simulink model "test_link"  (R2021a)
settings: Solver=ode15s  StartTime=0.0  StopTime=50  FixedStep=1  MaxStep=0.02  RelTol=1e-10
values from neighbouring files (symbols this model uses):
  waypoints = [0 1.5 0;         1 1.5 0 ... (first row only)    [manipulator.m]    (also in manipulatorsim.m = [0 1.5 0; 0.25 1.5 0)
  waypointVels = 0.01 *[ 0  1  0 ... (first row only)    [manipulator.m]    (also in manipulatorsim.m = 0.02 *[ 0  0.75  0;0.5 0 0)
  waytime = 0:6:30    [manipulator.m]    (also in manipulatorsim.m = 0:2:22)
libraries: robotmaniplib x1, robotcorelib x1
settings Model: Creator=Harish SG  LastModifiedBy=Harish SG
settings SolverCC: MaxOrder=2  MaxConsecutiveMinStep=2

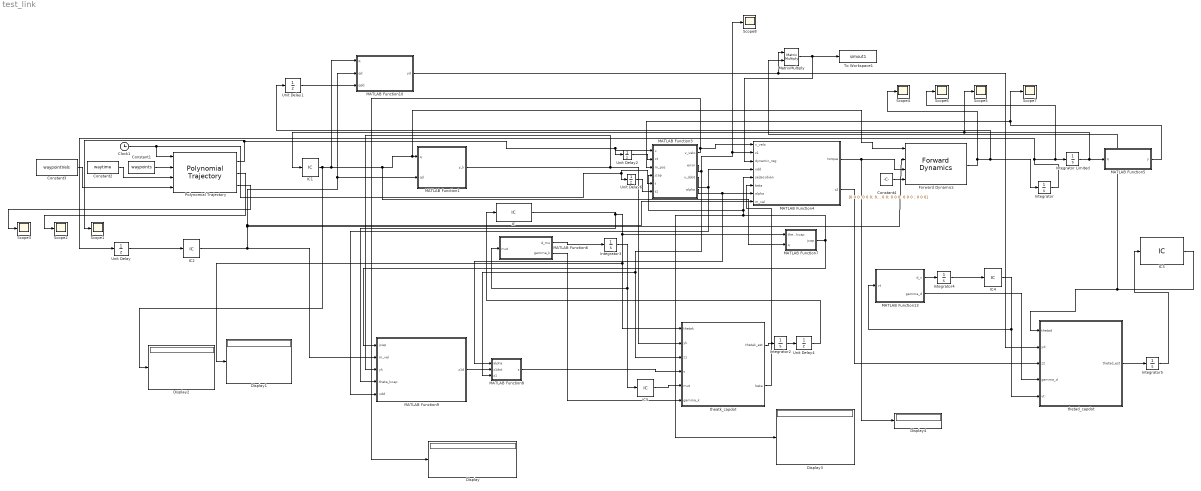
== system test_link ==
  " theatk_capdot" : MATLAB Function  TreatAsAtomicUnit=on
  Clock1 : Clock
  Constant1 : Constant  Value=waypoints
  Constant2 : Constant  Value=waytime
  Constant3 : Constant  Value=waypointVels
  Constant4 : Constant  Value=[0 0 0 ;0 0 0; 0 0 0; 0 0 0; 0 0 0 ; 0 0 0]
  Display{,1..4} (5 alike) : Display
  Forward Dynamics : robotmaniplib/Forward Dynamics  RigidBodyTree=planar_arm  SimulateUsing=Interpreted execution
  IC : InitialCondition  Value=[0.4;0.4;0.4;0.4]
  IC1 : InitialCondition  Value=[pi/3;pi/3]
  IC2 : InitialCondition  Value=[0;0]
  IC3 : InitialCondition  Value=|
      | [3.0000;0.7500;1.0830;0
      | ;3.0000
      | ;0.7500;0.4375
      | ;0]
  IC4 : InitialCondition  Value=[0.01;0.01;0.01;0.01;0.01;0.01;0.01;0.01]
  IC5 : InitialCondition  Value=[1;0.1;1;0.1]
  Integrator : Integrator  IgnoreLimit=on  ContinuousStateAttributes='acceleration'
  Integrator Limited : Integrator  LimitOutput=on  UpperSaturationLimit=1  LowerSaturationLimit=0
  Integrator{2..5} (4 alike) : Integrator
  MATLAB Function1 : MATLAB Function  TreatAsAtomicUnit=on
  MATLAB Function10 : MATLAB Function  TreatAsAtomicUnit=on
  MATLAB Function13 : MATLAB Function  TreatAsAtomicUnit=on
  MATLAB Function3 : MATLAB Function  TreatAsAtomicUnit=on
  MATLAB Function4 : MATLAB Function  TreatAsAtomicUnit=on
  MATLAB Function5 : MATLAB Function  TreatAsAtomicUnit=on
  MATLAB Function6 : MATLAB Function  TreatAsAtomicUnit=on
  MATLAB Function7 : MATLAB Function  TreatAsAtomicUnit=on
  MATLAB Function8 : MATLAB Function  TreatAsAtomicUnit=on
  MATLAB Function9 : MATLAB Function  TreatAsAtomicUnit=on
  MatrixMultiply : Product  Multiplication=Matrix(*)
  Polynomial Trajectory : robotcorelib/Polynomial Trajectory  WaypointSource=External  Waypoints=[ 0, 2, 1, 5, 0; -1, 3, 1, 4, 4 ]  TimePoints=[ 0, 1, 2, 3, 4 ]  TimeInterval=[ 1, 4 ]  Method=Cubic Polynomial  ParameterSource=External  VelocityBoundaryCondition=zeros( 2, 5 )  AccelerationBoundaryCondition=zeros( 2, 5 )  SimulateUsing=Interpreted execution
  Scope{1..8} (8 alike) : Scope
  To Workspace1 : ToWorkspace  VariableName=simout1  SaveFormat=Timeseries  SampleTime=-1
  Unit Delay{,1..2,4,6} (5 alike) : UnitDelay  SampleTime=-1  HasFrameUpgradeWarning=on
  thetad_capdot : MATLAB Function  TreatAsAtomicUnit=on
  wires:
  Clock1/1 -> Polynomial Trajectory/1, Unit Delay6/1, MATLAB Function3/5(t)
  Constant1/1 -> Polynomial Trajectory/2
  Constant2/1 -> Polynomial Trajectory/3
  Constant3/1 -> Polynomial Trajectory/4
  Polynomial Trajectory/1 -> Scope1/1, Unit Delay2/1, MATLAB Function3/1(x)
  Polynomial Trajectory/2 -> Scope2/1
  Polynomial Trajectory/3 -> Scope3/1
  MATLAB Function3/1(v_velo) -> Display/1, MATLAB Function4/1(v_velo)
  MATLAB Function4/1(torque) -> Display4/1, Forward Dynamics/3
  Constant4/1 -> Forward Dynamics/4
  Integrator Limited/1 -> IC1/1, Scope5/1, MATLAB Function5/1(q)
  MATLAB Function3/2(error) -> Scope8/1, MATLAB Function4/2(z1), MATLAB Function8/3(z1), " theatk_capdot"/3(z1)
  IC/1 -> MATLAB Function9/4(theta_kcap), MATLAB Function7/1(thetakcap), " theatk_capdot"/1(thetak), Display1/1
  MATLAB Function1/1(y_k) -> MATLAB Function9/3(yk), " theatk_capdot"/2(yk)
  " theatk_capdot"/1(thetak_est) -> Integrator2/1
  MATLAB Function6/1(d_mu) -> Integrator3/1
  MATLAB Function8/1(s) -> " theatk_capdot"/4(s)
  Integrator3/1 -> IC5/1, MATLAB Function6/1(mut)
  " theatk_capdot"/2(beta) -> MATLAB Function4/6(beta)
  MATLAB Function9/1(z1d) -> MATLAB Function8/2(z1dot)
  MATLAB Function3/3(x_ddot) -> MATLAB Function4/4(xdd), MATLAB Function9/5(xdd)
  MATLAB Function10/1(yd) -> thetad_capdot/2(yd), MatrixMultiply/1
  IC3/1 -> thetad_capdot/1(thetad), MatrixMultiply/2
  MATLAB Function4/2(z2) -> thetad_capdot/3(z2)
  MATLAB Function13/1(d_v) -> Integrator4/1
  Integrator4/1 -> IC4/1
  thetad_capdot/1(thetad_est) -> Integrator5/1
  MATLAB Function6/2(gamma_k) -> " theatk_capdot"/6(gamma_k)
  MATLAB Function13/2(gamma_d) -> thetad_capdot/4(gamma_d)
  Integrator/1 -> Unit Delay/1, Integrator Limited/1, Scope6/1
  Integrator2/1 -> Unit Delay4/1
  Unit Delay4/1 -> IC/1
  MATLAB Function5/1(y) -> Scope7/1, MATLAB Function3/3(m_pos)
  Unit Delay1/1 -> MATLAB Function10/3(qdd)
  MatrixMultiply/1 -> To Workspace1/1, MATLAB Function4/3(dynamic_reg)
  IC2/1 -> MATLAB Function9/2(m_vel), MATLAB Function1/2(qd), MATLAB Function10/2(qd), MATLAB Function4/8(m_vel), Forward Dynamics/2
  Unit Delay/1 -> IC2/1
  Integrator5/1 -> IC3/1
  MATLAB Function7/1(jcap) -> MATLAB Function9/1(jcap), Display3/1, MATLAB Function4/5(selJacobian), MATLAB Function3/4(jcap)
  IC1/1 -> Display2/1, MATLAB Function10/1(q), MATLAB Function7/2(q), Forward Dynamics/1, MATLAB Function1/1(q)
  Unit Delay2/1 -> MATLAB Function3/2(xt)
  Unit Delay6/1 -> MATLAB Function3/6(t1)
  IC4/1 -> MATLAB Function13/1(vt), thetad_capdot/5(vt)
  IC5/1 -> " theatk_capdot"/5(mut)
  Forward Dynamics/1 -> Scope4/1, Integrator/1, Unit Delay1/1
  MATLAB Function3/4(alpha) -> MATLAB Function8/1(alpha), MATLAB Function4/7(alpha)

== matlab function test_link/MATLAB Function9 ==
  data: jcap input; z1d output; m_vel input; yk input; theta_kcap input; xdd input
function z1d = z1d(jcap,m_vel,yk,theta_kcap,xdd)
a2 = 0.5; 
l1 = 0.25;
theta_k = [l1;a2;l1;a2];
theta_k_ = theta_k - theta_kcap; 
z1d = jcap*m_vel+yk*theta_k_-xdd;

== matlab function test_link/MATLAB Function10 ==
  data: q input; yd output; qd input; qdd input
function yd = yd(q,qd,qdd)
g = 0;
l1 = 0.25;l2 =0.25;a1 =0.5;a2=0.5;
 q1 = q(1);
 q2 = q(2);
 qd1 = qd(1);
 qd2 = qd(2);
 qdd1 = qdd(1);
 qdd2 = qdd(2);
 y11 = (l1^2)*qdd1 + l1*g*cos(q1);
 y12 = 2*l1*qdd1 +g*cos(q1);
 y13 = qdd1;
 y14 = 0;
 y15 = ((l1^2)+2*l1*l2*cos(q1)+(l2^2))*qdd1 + (l1*l2*cos(q2)+(l1^2))*qdd2 - (2*l1*l2*sin(q2)*qd1*qd2)- l1*l2*sin(q2)*(qd2^2) +l1*g*cos(q1)+l2*g*cos(q1+q2);
 y16 = (2*l1*cos(q1)+2*l2)*qdd1 + (l1*cos(q2)+2*l2)*qdd2 - 2*l1*sin(q1)*qd1*qd2 - l1*sin(q2)*(cos(q2)^2)+g*cos(q1+q2);
 y17 = qdd1+qdd2;
 y18 = 0;
 y21 =0; y22=0;y23=0;y24=0;y28=0;
 y27 = qdd1+qdd2;
 y25 = (2*l1*l2*cos(q2)+a2^2)*qdd1+ l2^2*qdd2+l1*l2*sin(q2)*(qd1)^2+l2*g*cos(q1+q2);
 y26 = (a1*cos(q2)+2*l2)*qdd1 + 2*l2*qdd2 +l1*sin(q2)*qd1^2+g*cos(q1+q2);
 yd = [y11,y12,y13,y14,y15,y16,y17,y18;...
     y21,y22,y23,y24,y25,y26,y27,y28];

== matlab function test_link/thetad_capdot ==
  data: thetad input; thetad_est output; yd input; z2 input; gamma_d input; vt input
function thetad_est = thetak_capdot(thetad,yd,z2,gamma_d,vt)

ydtrans = yd';

thetad_est =gamma_d*(ydtrans*z2) - diag(vt) * thetad;

== matlab function test_link/MATLAB Function13 ==
  data: vt input; d_v output; gamma_d output
function [d_v,gamma_d] = d_v(vt)
a =3;
gamma_d = a*eye(8);
ingammad = inv(gamma_d);
d_v = -(ingammad*vt);

== matlab function test_link/MATLAB Function1 ==
  data: q input; y_k output; qd input
function y_k = yk(q,qd)
     q1 = q(1);
     q2 = q(2);
     qd1 = qd(1);
     qd2 = qd(2);
      y_k = [-sin(q1)*qd1, -sin(q1+q2)*(qd1+qd2),0,0;...
     0,0,cos(q1)*qd1, cos(q1+q2)*(qd1+qd2)];

== matlab function test_link/ theatk_capdot ==
  data: thetak input; thetak_est output; yk input; z1 input; s input; mut input; beta output; gamma_k input
function [thetak_est,beta] = thetak_capdot(thetak,yk,z1,s,mut,gamma_k)
beta = 10;

yktrans = yk';


thetak_est = gamma_k*((yktrans*z1) + (2*beta*yktrans*s))- diag(mut)* thetak;

== matlab function test_link/MATLAB Function3 ==
  data: x input; xt input; v_velo output; m_pos input; error output; x_ddot output; jcap input; t input; t1 input; alpha output
function [v_velo,error,x_ddot,alpha] = virtControl(x,xt,m_pos,jcap,t,t1)
alpha = 1;
if t <= 0 
    x_ddot = [0;0];
else
    xdd= differt(x,xt,t,t1);
    x_ddot = xdd(1:2,:);
end
    ijcap = inv(jcap);
error = m_pos - x(1:2,:);
eie = x_ddot - (alpha*error);
v_velo = ijcap*eie;
function xdd = differt(x,xt,t,t1)
    dx = x-xt;
    dt = t-t1;
    xdd = dx/dt;
end
end

== matlab function test_link/MATLAB Function4 ==
  data: v_velo input; z1 input; dynamic_reg input; xdd input; torque output; selJacobian input; beta input; alpha input; z2 output; m_vel input
function [torque,z2] = subSysttwo(v_velo,z1,dynamic_reg,xdd,selJacobian,beta,alpha,m_vel)
eta =100;
scap = selJacobian*m_vel-xdd+alpha*z1(1:2,:); 
z2 = m_vel - v_velo;
torque =  -((selJacobian')*z1(1:2,:)) -(beta*(selJacobian')*scap) - (eta*z2)+dynamic_reg ;

 %v_velo is the virtual joint control
 %m_vel is the measureed joint velocity
 %homeconfig is the measure joint angle
 %qdd is the measured acceleration

== matlab function test_link/MATLAB Function5 ==
  data: q input; y output
function y = forwarDynamics(q)
 q1 = q(1);
 q2 = q(2);
 l1 = 1; l2 =1;
 y = [ l1*cos(q1) + l2*cos(q1+q2) ;...
          l1*sin(q1) + l2*sin(q1+q2) ];

== matlab function test_link/MATLAB Function6 ==
  data: mut input; d_mu output; gamma_k output
function [d_mu,gamma_k] = d_mu(mut)

gamma_k = 2*eye(4);
ingammak = inv(gamma_k);
d_mu = -(ingammak*mut);

== matlab function test_link/MATLAB Function7 ==
  data: thetakcap input; jcap output; q input
function jcap = Jcap(thetakcap,q)
a1 = thetakcap(1);
a2 = thetakcap(2);
q1 =q(1);
q2 =q(2);
jcap = [((-a1*sin(q1))-(a2*sin(q1+q2))), -(a2*sin(q1+q2)); 
    ((a1*cos(q1))+(a2*cos(q1+q2))), (a2*cos(q1+q2))];

== matlab function test_link/MATLAB Function8 ==
  data: alpha input; s output; z1dot input; z1 input
function s = s(alpha,z1dot,z1)

s = z1dot+(alpha*z1);
